simulink model "Cooperative_Localization_05_New2"  (R2016b)
settings: Solver=ode45  StartTime=0.0  StopTime=200  RelTol=1e-3  EnableMultiTasking=on
InitFcn:
  | Const_Coop_Local_05
undefined symbols (not defined in the file): alpha, AN, B, B_pseudo_inverse, BBT_inv, BN, D, Delta_form, Gama0, gamma0, gamma_0, gamma_1, H, K, k0_est, k1, k1_est, k2, KI, Ki_1, Ki_2, Ki_3, Ki_4, lambda, m_cont, Mb, Mu, n, N, n_cont, Observer_Gain, P_struct, Q, Q1, R, Rho1, Rho_0, rho_0, rho_1, t_cont, U_dot0_M
(part 1 of 3)
settings Model: SimulationMode=rapid-accelerator  Creator=hp  LastModifiedBy=hp
settings DataIOCC: LimitDataPoints=on  SaveFormat=Array
settings OptimizationCC: LifeSpan=inf
settings DebuggingCC: UnderspecifiedInitializationDetection=Classic  MergeDetectMultiDrivingBlocksExec=none  SolverPrmCheckMsg=warning  SFUnexpectedBacktrackingDiag=warning  SFNoUnconditionalDefaultTransitionDiag=warning  SFExecutionAtInitializationDiag=none
settings HardwareCC: ProdBitPerPointer=32  ProdBitPerSizeT=32  ProdBitPerPtrDiffT=32  ProdLargestAtomicFloat=None  ProdIntDivRoundTo=Undefined  ProdEndianess=Unspecified  ProdWordSize=32  ProdHWDeviceType=32-bit Generic
settings ModelReferenceCC: PropagateSignalLabelsOutOfModel=off
settings GRTTargetCC: TargetLangStandard=C89/C90 (ANSI)  GeneratePreprocessorConditionals=Disable all
settings ConfigComp: CovMetricSettings=dw  CovHtmlReporting=on  CovSaveCumulativeToWorkspaceVar=on  CovSaveSingleToWorkspaceVar=on  CovExternalEMLEnable=off

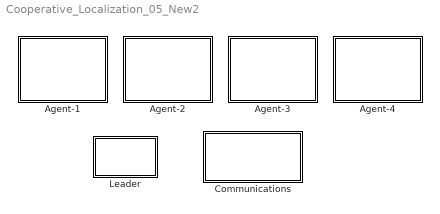
== system Cooperative_Localization_05_New2 ==
  Agent-1 : Subsystem
  Agent-2 : Subsystem
  Agent-3 : Subsystem
  Agent-4 : Subsystem
  Communications : Subsystem
  Leader : Subsystem

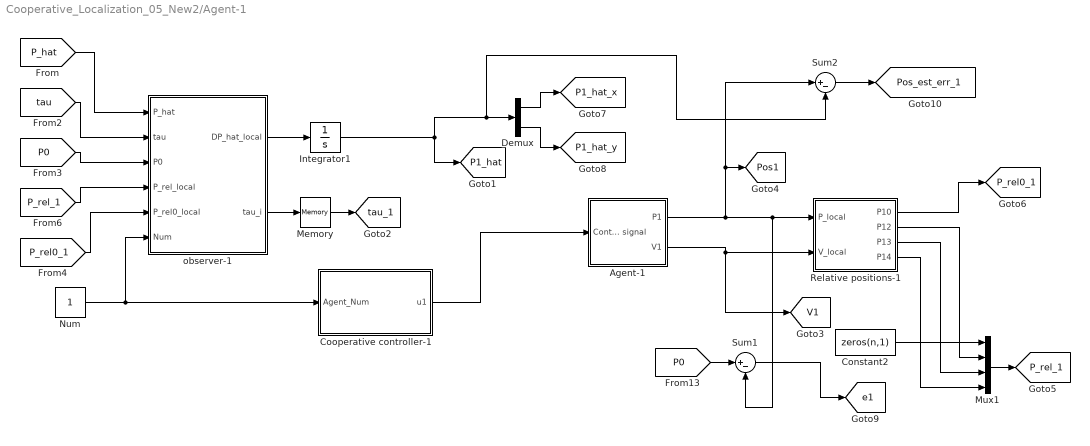
== system Cooperative_Localization_05_New2/Agent-1 ==
  Agent-1 : Subsystem
  Constant2 : Constant  Value=zeros(n,1)
  Cooperative controller-1 : Subsystem
  Demux : Demux  Outputs=2
  Integrator1 : Integrator  InitialCondition=zeros(n,1)
  Memory : Memory  X0=zeros(n,1)
  Mux1 : Mux
  Num : Constant
  Relative positions-1 : Subsystem
  Sum1 : Sum  Inputs=|+-
  Sum2 : Sum  Inputs=|+-
  observer-1 : MATLAB Function  TreatAsAtomicUnit=on
  tag scope: P1_hat=global, P1_hat_x=global, P1_hat_y=global, P_rel0_1=global, P_rel_1=global, Pos1=global, Pos_est_err_1=global, V1=global, e1=global, tau_1=global
  wires:
  observer-1/1(DP_hat_local) -> Integrator1/1
  Integrator1/1 -> [P1_hat], Sum2/2, Demux/1
  [P_hat] -> observer-1/1(P_hat)
  [tau] -> observer-1/2(tau)
  [P0] -> observer-1/3(P0)
  [P_rel0_1] -> observer-1/5(P_rel0_local)
  observer-1/2(tau_i) -> Memory/1
  [P_rel_1] -> observer-1/4(P_rel_local)
  Memory/1 -> [tau_1]
  Agent-1/2(V1) -> Relative positions-1/2(V_local), [V1]
  Agent-1/1(P1) -> Relative positions-1/1(P_local), Sum1/2, [Pos1], Sum2/1
  Mux1/1 -> [P_rel_1]
  Relative positions-1/1(P10) -> [P_rel0_1]
  Demux/1 -> [P1_hat_x]
  Demux/2 -> [P1_hat_y]
  Constant2/1 -> Mux1/1
  Relative positions-1/2(P12) -> Mux1/2
  Relative positions-1/3(P13) -> Mux1/3
  Relative positions-1/4(P14) -> Mux1/4
  Sum1/1 -> [e1]
  Sum2/1 -> [Pos_est_err_1]
  [P0] -> Sum1/1
  Num/1 -> Cooperative controller-1/1(Agent_Num), observer-1/6(Num)
  Cooperative controller-1/1(u1) -> Agent-1/1(Control signal)

== system Cooperative_Localization_05_New2/Agent-2 ==
  Agent-2 : Subsystem
  Constant2 : Constant  Value=zeros(n,1)
  Cooperative controller-2 : Subsystem
  Demux : Demux  Outputs=2
  Integrator1 : Integrator  InitialCondition=zeros(n,1)
  Memory : Memory  X0=zeros(n,1)
  Mux1 : Mux
  Num : Constant  Value=2
  Relative positions-2 : Subsystem
  Sum1 : Sum  Inputs=|+-
  Sum2 : Sum  Inputs=|+-
  observer-1 : MATLAB Function  TreatAsAtomicUnit=on
  tag scope: P2_hat=global, P2_hat_x=global, P2_hat_y=global, P_rel0_2=global, P_rel_2=global, Pos2=global, Pos_est_err_2=global, V2=global, e2=global, tau_2=global
  wires:
  Relative positions-2/4(P24) -> Mux1/4
  Relative positions-2/3(P23) -> Mux1/3
  Demux/2 -> [P2_hat_y]
  Demux/1 -> [P2_hat_x]
  Relative positions-2/1(P20) -> [P_rel0_2]
  Mux1/1 -> [P_rel_2]
  Agent-2/2(V2) -> Relative positions-2/2(V_local), [V2]
  Cooperative controller-2/1(u2) -> Agent-2/1(Control signal)
  Memory/1 -> [tau_2]
  [P_rel_2] -> observer-1/4(P_rel_local)
  observer-1/2(tau_i) -> Memory/1
  [P_rel0_2] -> observer-1/5(P_rel0_local)
  [P0] -> observer-1/3(P0)
  [tau] -> observer-1/2(tau)
  [P_hat] -> observer-1/1(P_hat)
  observer-1/1(DP_hat_local) -> Integrator1/1
  Constant2/1 -> Mux1/2
  Relative positions-2/2(P21) -> Mux1/1
  Sum1/1 -> [e2]
  Integrator1/1 -> Sum2/2, Demux/1, [P2_hat]
  Agent-2/1(P2) -> Sum2/1, [Pos2], Relative positions-2/1(P_local), Sum1/2
  Sum2/1 -> [Pos_est_err_2]
  Num/1 -> Cooperative controller-2/1(Agent_Num), observer-1/6(Num)
  [P0] -> Sum1/1

== system Cooperative_Localization_05_New2/Agent-3 ==
  Agent-3 : Subsystem
  Constant2 : Constant  Value=zeros(n,1)
  Cooperative controller-3 : Subsystem
  Demux : Demux  Outputs=2
  Integrator1 : Integrator  InitialCondition=zeros(n,1)
  Memory : Memory  X0=zeros(n,1)
  Mux1 : Mux
  Num : Constant  Value=3
  Relative positions-3 : Subsystem
  Sum1 : Sum  Inputs=|+-
  Sum2 : Sum  Inputs=|+-
  observer-1 : MATLAB Function  TreatAsAtomicUnit=on
  tag scope: P3_hat=global, P3_hat_x=global, P3_hat_y=global, P_rel0_3=global, P_rel_3=global, Pos3=global, Pos_est_err_3=global, V3=global, e3=global, tau_3=global
  wires:
  observer-1/1(DP_hat_local) -> Integrator1/1
  [P_hat] -> observer-1/1(P_hat)
  [tau] -> observer-1/2(tau)
  [P0] -> observer-1/3(P0)
  [P_rel0_3] -> observer-1/5(P_rel0_local)
  observer-1/2(tau_i) -> Memory/1
  [P_rel_3] -> observer-1/4(P_rel_local)
  Memory/1 -> [tau_3]
  Agent-3/2(V3) -> Relative positions-3/2(V_local), [V3]
  Mux1/1 -> [P_rel_3]
  Relative positions-3/1(P30) -> [P_rel0_3]
  Demux/1 -> [P3_hat_x]
  Demux/2 -> [P3_hat_y]
  Constant2/1 -> Mux1/3
  Relative positions-3/2(P31) -> Mux1/1
  Relative positions-3/3(P32) -> Mux1/2
  Relative positions-3/4(P34) -> Mux1/4
  Sum1/1 -> [e3]
  Integrator1/1 -> [P3_hat], Sum2/2, Demux/1
  Agent-3/1(P3) -> Relative positions-3/1(P_local), Sum1/2, Sum2/1, [Pos3]
  Sum2/1 -> [Pos_est_err_3]
  Num/1 -> Cooperative controller-3/1(Agent_Num), observer-1/6(Num)
  [P0] -> Sum1/1
  Cooperative controller-3/1(u3) -> Agent-3/1(Control signal)

== system Cooperative_Localization_05_New2/Agent-4 ==
  Agent-4 : Subsystem
  Constant2 : Constant  Value=zeros(n,1)
  Cooperative controller-4 : Subsystem
  Demux : Demux  Outputs=2
  Integrator1 : Integrator  InitialCondition=zeros(n,1)
  Memory : Memory  X0=zeros(n,1)
  Mux1 : Mux
  Num : Constant  Value=4
  Relative positions-4 : Subsystem
  Sum1 : Sum  Inputs=|+-
  Sum2 : Sum  Inputs=|+-
  observer-1 : MATLAB Function  TreatAsAtomicUnit=on
  tag scope: P4_hat=global, P4_hat_x=global, P4_hat_y=global, P_rel0_4=global, P_rel_4=global, Pos4=global, Pos_est_err_4=global, V4=global, e4=global, tau_4=global
  wires:
  Demux/2 -> [P4_hat_y]
  Demux/1 -> [P4_hat_x]
  Relative positions-4/1(P40) -> [P_rel0_4]
  Mux1/1 -> [P_rel_4]
  Agent-4/2(V4) -> Relative positions-4/2(V_local), [V4]
  Memory/1 -> [tau_4]
  [P_rel_4] -> observer-1/4(P_rel_local)
  observer-1/2(tau_i) -> Memory/1
  [P_rel0_4] -> observer-1/5(P_rel0_local)
  [P0] -> observer-1/3(P0)
  [tau] -> observer-1/2(tau)
  [P_hat] -> observer-1/1(P_hat)
  observer-1/1(DP_hat_local) -> Integrator1/1
  Constant2/1 -> Mux1/4
  Relative positions-4/2(P41) -> Mux1/1
  Relative positions-4/3(P42) -> Mux1/2
  Relative positions-4/4(P43) -> Mux1/3
  Sum1/1 -> [e4]
  Integrator1/1 -> Sum2/2, Demux/1, [P4_hat]
  Agent-4/1(P4) -> Sum2/1, [Pos4], Relative positions-4/1(P_local), Sum1/2
  Sum2/1 -> [Pos_est_err_4]
  Num/1 -> Cooperative controller-4/1(Agent_Num), observer-1/6(Num)
  [P0] -> Sum1/1
  Cooperative controller-4/1(u4) -> Agent-4/1(Control signal)

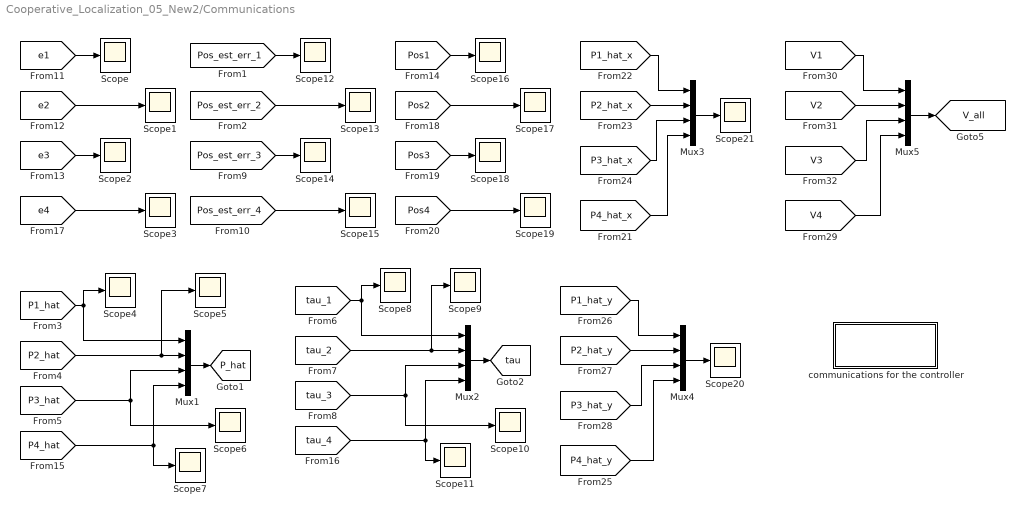
== system Cooperative_Localization_05_New2/Communications ==
  Mux{1..5} (5 alike) : Mux
  Scope{,1..21} (22 alike) : Scope
  communications for the controller : Subsystem
  tag scope: P_hat=global, V_all=global, tau=global
  wires:
  [P1_hat] -> Scope4/1, Mux1/1
  [P2_hat] -> Scope5/1, Mux1/2
  [P3_hat] -> Mux1/3, Scope6/1
  Mux1/1 -> [P_hat]
  [tau_1] -> Scope8/1, Mux2/1
  [tau_2] -> Scope9/1, Mux2/2
  [tau_3] -> Mux2/3, Scope10/1
  Mux2/1 -> [tau]
  [P4_hat] -> Scope7/1, Mux1/4
  [tau_4] -> Scope11/1, Mux2/4
  [e1] -> Scope/1
  [e2] -> Scope1/1
  [e3] -> Scope2/1
  [e4] -> Scope3/1
  [Pos_est_err_1] -> Scope12/1
  [Pos_est_err_2] -> Scope13/1
  [Pos_est_err_3] -> Scope14/1
  [Pos_est_err_4] -> Scope15/1
  [Pos1] -> Scope16/1
  [Pos2] -> Scope17/1
  [Pos3] -> Scope18/1
  [Pos4] -> Scope19/1
  [P1_hat_x] -> Mux3/1
  [P2_hat_x] -> Mux3/2
  [P3_hat_x] -> Mux3/3
  Mux3/1 -> Scope21/1
  [P4_hat_x] -> Mux3/4
  [P1_hat_y] -> Mux4/1
  [P2_hat_y] -> Mux4/2
  [P3_hat_y] -> Mux4/3
  Mux4/1 -> Scope20/1
  [P4_hat_y] -> Mux4/4
  [V1] -> Mux5/1
  [V2] -> Mux5/2
  [V3] -> Mux5/3
  Mux5/1 -> [V_all]
  [V4] -> Mux5/4

== system Cooperative_Localization_05_New2/Leader ==
  Agent-0 : Subsystem
  Ali : Subsystem
  Constant4 : Constant  Value=2
  Constant5 : Constant
  Controller interpreter : MATLAB Function  TreatAsAtomicUnit=on
  Mux1 : Mux  Inputs=2
  Mux2 : Mux  Inputs=2
  Scope{,1..4} (5 alike) : Scope
  Sine Wave : Sin  Amplitude=4  Frequency=0.1  SampleTime=0
  Sine Wave1 : Sin  Amplitude=6  Frequency=0.05  SampleTime=0
  Sum : Sum  Inputs=|+-
  Transfer Fcn : TransferFcn  Denominator=[10 1]
  Transfer Fcn1 : TransferFcn  Denominator=[10 1]
  formation of the leader : Constant  Value=zeros(n_cont,1)
  tag scope: P0=global, U0=global, V0=global, Z0=global
  wires:
  Sum/1 -> [Z0]
  formation of the leader/1 -> Sum/2
  Controller interpreter/1(u) -> Agent-0/1(Control signal), Mux2/2
  Ali/1(u) -> Scope/1, Controller interpreter/1(U)
  Mux1/1 -> Ali/2(xd), Scope4/1
  Constant4/1 -> Transfer Fcn/1
  Constant5/1 -> Transfer Fcn1/1
  Agent-0/2(P0) -> [P0], Scope1/1
  Mux2/1 -> [U0]
  Agent-0/1(X0) -> Ali/1(x), Scope2/1, Sum/1
  Agent-0/3(V0) -> Scope3/1, Mux2/1, [V0]
  Sine Wave/1 -> Mux1/1
  Sine Wave1/1 -> Mux1/2

== system Cooperative_Localization_05_New2/Agent-1/Agent-1 ==
  Control signal : Inport
  Clock : Clock
  Demux : Demux
  Demux1 : Demux  Outputs=2
  Integrator : Integrator  InitialCondition=[0;0;0;0]
  MATLAB Function : MATLAB Function  TreatAsAtomicUnit=on
  Memory1 : Memory  X0=zeros(2,1)
  Memory4 : Memory  X0=zeros(2,1)
  Mux : Mux  Inputs=2
  Mux1 : Mux  Inputs=2
  P1 : Outport
  V1 : Outport  Port=2
  wires:
  MATLAB Function/1(out) -> Integrator/1
  Integrator/1 -> Demux/1
  Mux/1 -> Memory4/1
  Mux1/1 -> Memory1/1
  Control signal/1 -> Demux1/1
  Demux1/1 -> MATLAB Function/5(Ax)
  Demux1/2 -> MATLAB Function/6(Ay)
  Memory4/1 -> P1/1
  Memory1/1 -> V1/1
  Demux/3 -> MATLAB Function/3(Vx), Mux1/1
  Demux/4 -> MATLAB Function/4(Vy), Mux1/2
  Demux/1 -> MATLAB Function/1(Px), Mux/1
  Demux/2 -> MATLAB Function/2(Py), Mux/2
  Clock/1 -> MATLAB Function/7(t)

== system Cooperative_Localization_05_New2/Agent-1/Cooperative controller-1 ==
  Agent_Num : Inport
  Choosing real control variables : MATLAB Function  TreatAsAtomicUnit=on
  Decenteralized Cooperaive Controller #1 : Subsystem
  Module to compute Consensus Error #1 : MATLAB Function  TreatAsAtomicUnit=on
  Mux : Mux  Inputs=2
  Variable change : MATLAB Function  TreatAsAtomicUnit=on
  u1 : Outport
  tag scope: E1_Cont=global, X1_Cont=global
  wires:
  Agent_Num/1 -> Module to compute Consensus Error #1/6(Agent_Num), Decenteralized Cooperaive Controller #1/1(Agent #)
  Decenteralized Cooperaive Controller #1/1(U1) -> Variable change/1(U), Choosing real control variables/1(U)
  [P_rel0_1] -> Module to compute Consensus Error #1/2(P_rel0)
  Module to compute Consensus Error #1/1(Ep) -> [E1_Cont]
  [P_rel_1] -> Module to compute Consensus Error #1/1(P_rel_all)
  Choosing real control variables/1(u) -> u1/1
  Variable change/1(X_mod) -> [X1_Cont]
  Mux/1 -> Variable change/2(X)
  [P1_hat] -> Mux/1
  [V1] -> Mux/2
  [V1] -> Module to compute Consensus Error #1/3(V_loc)
  [V0] -> Module to compute Consensus Error #1/4(V0)
  [V_all] -> Module to compute Consensus Error #1/5(V_all)

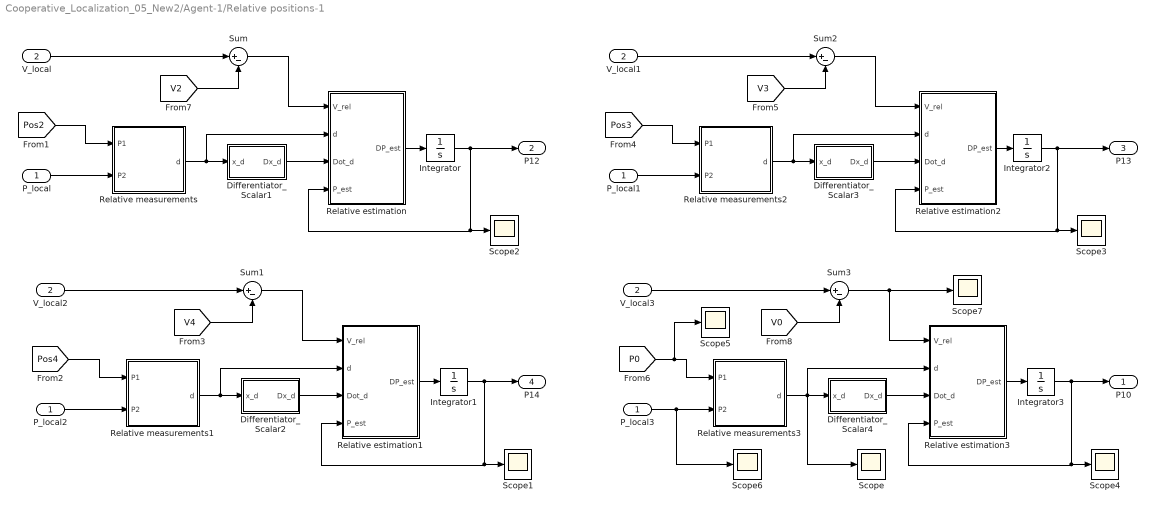
== system Cooperative_Localization_05_New2/Agent-1/Relative positions-1 ==
  P_local : Inport
  V_local : Inport  Port=2
  Differentiator_Scalar1 : Subsystem
  Differentiator_Scalar2 : Subsystem
  Differentiator_Scalar3 : Subsystem
  Differentiator_Scalar4 : Subsystem
  Integrator{,1..3} (4 alike) : Integrator  InitialCondition=zeros(2,1)
  P_local1 : InportShadow
  P_local2 : InportShadow
  P_local3 : InportShadow
  Relative estimation : MATLAB Function  TreatAsAtomicUnit=on
  Relative estimation1 : MATLAB Function  TreatAsAtomicUnit=on
  Relative estimation2 : MATLAB Function  TreatAsAtomicUnit=on
  Relative estimation3 : MATLAB Function  TreatAsAtomicUnit=on
  Relative measurements : MATLAB Function  TreatAsAtomicUnit=on
  Relative measurements1 : MATLAB Function  TreatAsAtomicUnit=on
  Relative measurements2 : MATLAB Function  TreatAsAtomicUnit=on
  Relative measurements3 : MATLAB Function  TreatAsAtomicUnit=on
  Scope{,1..7} (8 alike) : Scope
  Sum{,1..3} (4 alike) : Sum  Inputs=|+-
  V_local1 : InportShadow  Port=2
  V_local2 : InportShadow  Port=2
  V_local3 : InportShadow  Port=2
  P10 : Outport
  P12 : Outport  Port=2
  P13 : Outport  Port=3
  P14 : Outport  Port=4
  wires:
  Relative measurements/1(d) -> Relative estimation/2(d), Differentiator_Scalar1/1(x_d)
  Differentiator_Scalar1/1(Dx_d) -> Relative estimation/3(Dot_d)
  Relative estimation/1(DP_est) -> Integrator/1
  Integrator/1 -> P12/1, Scope2/1, Relative estimation/4(P_est)
  P_local/1 -> Relative measurements/2(P2)
  V_local/1 -> Sum/1
  Sum/1 -> Relative estimation/1(V_rel)
  [V2] -> Sum/2
  [Pos2] -> Relative measurements/1(P1)
  Relative measurements1/1(d) -> Relative estimation1/2(d), Differentiator_Scalar2/1(x_d)
  Differentiator_Scalar2/1(Dx_d) -> Relative estimation1/3(Dot_d)
  Relative estimation1/1(DP_est) -> Integrator1/1
  Integrator1/1 -> P14/1, Relative estimation1/4(P_est), Scope1/1
  P_local2/1 -> Relative measurements1/2(P2)
  V_local2/1 -> Sum1/1
  Sum1/1 -> Relative estimation1/1(V_rel)
  [V4] -> Sum1/2
  [Pos4] -> Relative measurements1/1(P1)
  Relative measurements2/1(d) -> Relative estimation2/2(d), Differentiator_Scalar3/1(x_d)
  Differentiator_Scalar3/1(Dx_d) -> Relative estimation2/3(Dot_d)
  Relative estimation2/1(DP_est) -> Integrator2/1
  Integrator2/1 -> P13/1, Relative estimation2/4(P_est), Scope3/1
  P_local1/1 -> Relative measurements2/2(P2)
  V_local1/1 -> Sum2/1
  Sum2/1 -> Relative estimation2/1(V_rel)
  [V3] -> Sum2/2
  [Pos3] -> Relative measurements2/1(P1)
  Relative measurements3/1(d) -> Scope/1, Relative estimation3/2(d), Differentiator_Scalar4/1(x_d)
  Differentiator_Scalar4/1(Dx_d) -> Relative estimation3/3(Dot_d)
  Relative estimation3/1(DP_est) -> Integrator3/1
  Integrator3/1 -> P10/1, Relative estimation3/4(P_est), Scope4/1
  P_local3/1 -> Scope6/1, Relative measurements3/2(P2)
  V_local3/1 -> Sum3/1
  Sum3/1 -> Scope7/1, Relative estimation3/1(V_rel)
  [V0] -> Sum3/2
  [P0] -> Scope5/1, Relative measurements3/1(P1)

== system Cooperative_Localization_05_New2/Agent-2/Agent-2 ==
  Control signal : Inport
  Clock : Clock
  Demux : Demux
  Demux1 : Demux  Outputs=2
  Integrator : Integrator  InitialCondition=[0;0;0;0]
  MATLAB Function : MATLAB Function  TreatAsAtomicUnit=on
  Memory1 : Memory  X0=zeros(2,1)
  Memory4 : Memory  X0=zeros(2,1)
  Mux : Mux  Inputs=2
  Mux1 : Mux  Inputs=2
  P2 : Outport
  V2 : Outport  Port=2
  wires:
  Demux/2 -> MATLAB Function/2(Py), Mux/2
  Demux/1 -> MATLAB Function/1(Px), Mux/1
  Demux/4 -> MATLAB Function/4(Vy), Mux1/2
  Demux/3 -> MATLAB Function/3(Vx), Mux1/1
  Memory1/1 -> V2/1
  Memory4/1 -> P2/1
  Demux1/2 -> MATLAB Function/6(Ay)
  Demux1/1 -> MATLAB Function/5(Ax)
  Control signal/1 -> Demux1/1
  Mux1/1 -> Memory1/1
  Mux/1 -> Memory4/1
  Integrator/1 -> Demux/1
  MATLAB Function/1(out) -> Integrator/1
  Clock/1 -> MATLAB Function/7(t)

== system Cooperative_Localization_05_New2/Agent-2/Cooperative controller-2 ==
  Agent_Num : Inport
  Choosing real control variables : MATLAB Function  TreatAsAtomicUnit=on
  Decenteralized Cooperaive Controller #2 : Subsystem
  Module to compute Consensus Error #2 : MATLAB Function  TreatAsAtomicUnit=on
  Mux : Mux  Inputs=2
  Variable change : MATLAB Function  TreatAsAtomicUnit=on
  u2 : Outport
  tag scope: E2_Cont=global, X2_Cont=global
  wires:
  Agent_Num/1 -> Module to compute Consensus Error #2/6(Agent_Num), Decenteralized Cooperaive Controller #2/1(Agent #)
  Decenteralized Cooperaive Controller #2/1(U2) -> Variable change/1(U), Choosing real control variables/1(U)
  [P_rel0_2] -> Module to compute Consensus Error #2/2(P_rel0)
  Module to compute Consensus Error #2/1(Ep) -> [E2_Cont]
  [P_rel_2] -> Module to compute Consensus Error #2/1(P_rel_all)
  Choosing real control variables/1(u) -> u2/1
  Variable change/1(X_mod) -> [X2_Cont]
  Mux/1 -> Variable change/2(X)
  [P2_hat] -> Mux/1
  [V2] -> Mux/2
  [V2] -> Module to compute Consensus Error #2/3(V_loc)
  [V0] -> Module to compute Consensus Error #2/4(V0)
  [V_all] -> Module to compute Consensus Error #2/5(V_all)

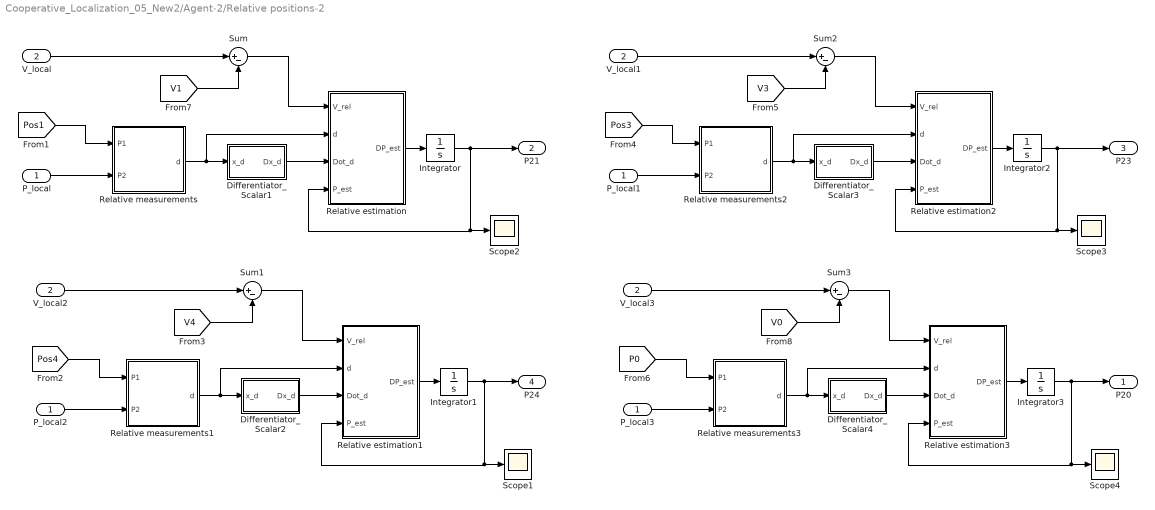
== system Cooperative_Localization_05_New2/Agent-2/Relative positions-2 ==
  P_local : Inport
  V_local : Inport  Port=2
  Differentiator_Scalar1 : Subsystem
  Differentiator_Scalar2 : Subsystem
  Differentiator_Scalar3 : Subsystem
  Differentiator_Scalar4 : Subsystem
  Integrator{,1..3} (4 alike) : Integrator  InitialCondition=zeros(2,1)
  P_local1 : InportShadow
  P_local2 : InportShadow
  P_local3 : InportShadow
  Relative estimation : MATLAB Function  TreatAsAtomicUnit=on
  Relative estimation1 : MATLAB Function  TreatAsAtomicUnit=on
  Relative estimation2 : MATLAB Function  TreatAsAtomicUnit=on
  Relative estimation3 : MATLAB Function  TreatAsAtomicUnit=on
  Relative measurements : MATLAB Function  TreatAsAtomicUnit=on
  Relative measurements1 : MATLAB Function  TreatAsAtomicUnit=on
  Relative measurements2 : MATLAB Function  TreatAsAtomicUnit=on
  Relative measurements3 : MATLAB Function  TreatAsAtomicUnit=on
  Scope{1..4} (4 alike) : Scope
  Sum{,1..3} (4 alike) : Sum  Inputs=|+-
  V_local1 : InportShadow  Port=2
  V_local2 : InportShadow  Port=2
  V_local3 : InportShadow  Port=2
  P20 : Outport
  P21 : Outport  Port=2
  P23 : Outport  Port=3
  P24 : Outport  Port=4
  wires:
  [P0] -> Relative measurements3/1(P1)
  [V0] -> Sum3/2
  Sum3/1 -> Relative estimation3/1(V_rel)
  V_local3/1 -> Sum3/1
  P_local3/1 -> Relative measurements3/2(P2)
  Integrator3/1 -> Relative estimation3/4(P_est), Scope4/1, P20/1
  Relative estimation3/1(DP_est) -> Integrator3/1
  Differentiator_Scalar4/1(Dx_d) -> Relative estimation3/3(Dot_d)
  Relative measurements3/1(d) -> Relative estimation3/2(d), Differentiator_Scalar4/1(x_d)
  [Pos3] -> Relative measurements2/1(P1)
  [V3] -> Sum2/2
  Sum2/1 -> Relative estimation2/1(V_rel)
  V_local1/1 -> Sum2/1
  P_local1/1 -> Relative measurements2/2(P2)
  Integrator2/1 -> Relative estimation2/4(P_est), Scope3/1, P23/1
  Relative estimation2/1(DP_est) -> Integrator2/1
  Differentiator_Scalar3/1(Dx_d) -> Relative estimation2/3(Dot_d)
  Relative measurements2/1(d) -> Relative estimation2/2(d), Differentiator_Scalar3/1(x_d)
  [Pos4] -> Relative measurements1/1(P1)
  [V4] -> Sum1/2
  Sum1/1 -> Relative estimation1/1(V_rel)
  V_local2/1 -> Sum1/1
  P_local2/1 -> Relative measurements1/2(P2)
  Integrator1/1 -> Relative estimation1/4(P_est), Scope1/1, P24/1
  Relative estimation1/1(DP_est) -> Integrator1/1
  Differentiator_Scalar2/1(Dx_d) -> Relative estimation1/3(Dot_d)
  Relative measurements1/1(d) -> Relative estimation1/2(d), Differentiator_Scalar2/1(x_d)
  [Pos1] -> Relative measurements/1(P1)
  [V1] -> Sum/2
  Sum/1 -> Relative estimation/1(V_rel)
  V_local/1 -> Sum/1
  P_local/1 -> Relative measurements/2(P2)
  Integrator/1 -> Relative estimation/4(P_est), Scope2/1, P21/1
  Relative estimation/1(DP_est) -> Integrator/1
  Differentiator_Scalar1/1(Dx_d) -> Relative estimation/3(Dot_d)
  Relative measurements/1(d) -> Relative estimation/2(d), Differentiator_Scalar1/1(x_d)

== system Cooperative_Localization_05_New2/Agent-3/Agent-3 ==
  Control signal : Inport
  Clock : Clock
  Demux : Demux
  Demux1 : Demux  Outputs=2
  Integrator : Integrator  InitialCondition=[0;0;0;0]
  MATLAB Function : MATLAB Function  TreatAsAtomicUnit=on
  Memory1 : Memory  X0=zeros(2,1)
  Memory4 : Memory  X0=[0;0]
  Mux : Mux  Inputs=2
  Mux1 : Mux  Inputs=2
  P3 : Outport
  V3 : Outport  Port=2
  tag scope: Vx3=global, Vy3=global
  wires:
  MATLAB Function/1(out) -> Integrator/1
  Integrator/1 -> Demux/1
  Mux/1 -> Memory4/1
  Mux1/1 -> Memory1/1
  Control signal/1 -> Demux1/1
  Demux1/1 -> MATLAB Function/5(Ax)
  Demux1/2 -> MATLAB Function/6(Ay)
  Memory4/1 -> P3/1
  Memory1/1 -> V3/1
  Demux/3 -> MATLAB Function/3(Vx), [Vx3], Mux1/1
  Demux/4 -> MATLAB Function/4(Vy), [Vy3], Mux1/2
  Demux/1 -> MATLAB Function/1(Px), Mux/1
  Demux/2 -> MATLAB Function/2(Py), Mux/2
  Clock/1 -> MATLAB Function/7(t)

== system Cooperative_Localization_05_New2/Agent-3/Cooperative controller-3 ==
  Agent_Num : Inport
  Choosing real control variables : MATLAB Function  TreatAsAtomicUnit=on
  Decenteralized Cooperaive Controller #3 : Subsystem
  Module to compute Consensus Error #3 : MATLAB Function  TreatAsAtomicUnit=on
  Mux : Mux  Inputs=2
  Variable change : MATLAB Function  TreatAsAtomicUnit=on
  u3 : Outport
  tag scope: E3_Cont=global, X3_Cont=global
  wires:
  Agent_Num/1 -> Module to compute Consensus Error #3/6(Agent_Num), Decenteralized Cooperaive Controller #3/1(Agent #)
  Decenteralized Cooperaive Controller #3/1(U3) -> Variable change/1(U), Choosing real control variables/1(U)
  [P_rel0_3] -> Module to compute Consensus Error #3/2(P_rel0)
  Module to compute Consensus Error #3/1(Ep) -> [E3_Cont]
  [P_rel_3] -> Module to compute Consensus Error #3/1(P_rel_all)
  Choosing real control variables/1(u) -> u3/1
  Variable change/1(X_mod) -> [X3_Cont]
  Mux/1 -> Variable change/2(X)
  [P3_hat] -> Mux/1
  [V3] -> Mux/2
  [V3] -> Module to compute Consensus Error #3/3(V_loc)
  [V0] -> Module to compute Consensus Error #3/4(V0)
  [V_all] -> Module to compute Consensus Error #3/5(V_all)

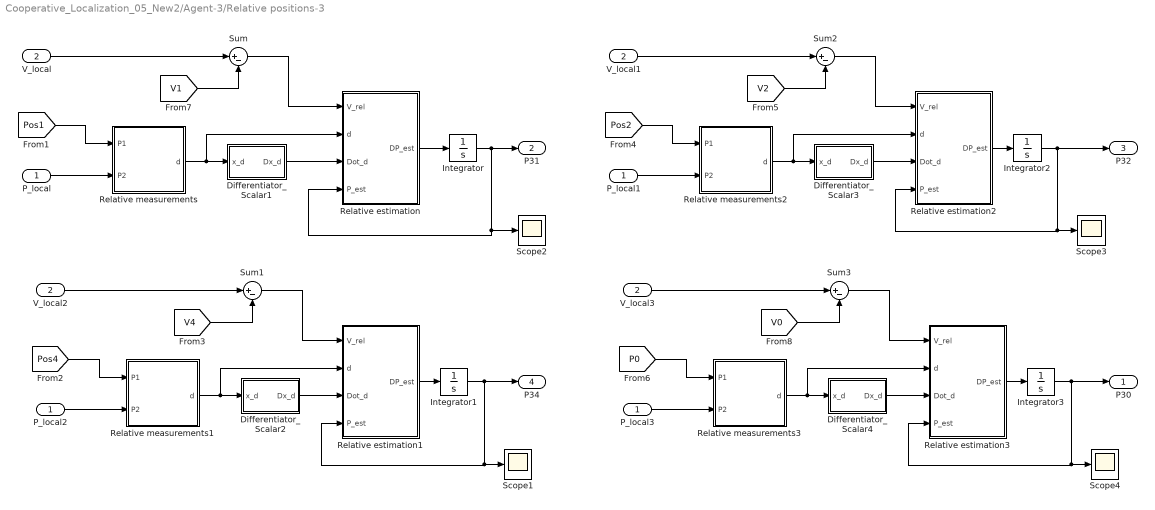
== system Cooperative_Localization_05_New2/Agent-3/Relative positions-3 ==
  P_local : Inport
  V_local : Inport  Port=2
  Differentiator_Scalar1 : Subsystem
  Differentiator_Scalar2 : Subsystem
  Differentiator_Scalar3 : Subsystem
  Differentiator_Scalar4 : Subsystem
  Integrator{,1..3} (4 alike) : Integrator  InitialCondition=zeros(2,1)
  P_local1 : InportShadow
  P_local2 : InportShadow
  P_local3 : InportShadow
  Relative estimation : MATLAB Function  TreatAsAtomicUnit=on
  Relative estimation1 : MATLAB Function  TreatAsAtomicUnit=on
  Relative estimation2 : MATLAB Function  TreatAsAtomicUnit=on
  Relative estimation3 : MATLAB Function  TreatAsAtomicUnit=on
  Relative measurements : MATLAB Function  TreatAsAtomicUnit=on
  Relative measurements1 : MATLAB Function  TreatAsAtomicUnit=on
  Relative measurements2 : MATLAB Function  TreatAsAtomicUnit=on
  Relative measurements3 : MATLAB Function  TreatAsAtomicUnit=on
  Scope{1..4} (4 alike) : Scope
  Sum{,1..3} (4 alike) : Sum  Inputs=|+-
  V_local1 : InportShadow  Port=2
  V_local2 : InportShadow  Port=2
  V_local3 : InportShadow  Port=2
  P30 : Outport
  P31 : Outport  Port=2
  P32 : Outport  Port=3
  P34 : Outport  Port=4
  wires:
  Relative measurements/1(d) -> Relative estimation/2(d), Differentiator_Scalar1/1(x_d)
  Differentiator_Scalar1/1(Dx_d) -> Relative estimation/3(Dot_d)
  Relative estimation/1(DP_est) -> Integrator/1
  Integrator/1 -> P31/1, Relative estimation/4(P_est), Scope2/1
  P_local/1 -> Relative measurements/2(P2)
  V_local/1 -> Sum/1
  Sum/1 -> Relative estimation/1(V_rel)
  [V1] -> Sum/2
  [Pos1] -> Relative measurements/1(P1)
  Relative measurements1/1(d) -> Relative estimation1/2(d), Differentiator_Scalar2/1(x_d)
  Differentiator_Scalar2/1(Dx_d) -> Relative estimation1/3(Dot_d)
  Relative estimation1/1(DP_est) -> Integrator1/1
  Integrator1/1 -> P34/1, Relative estimation1/4(P_est), Scope1/1
  P_local2/1 -> Relative measurements1/2(P2)
  V_local2/1 -> Sum1/1
  Sum1/1 -> Relative estimation1/1(V_rel)
  [V4] -> Sum1/2
  [Pos4] -> Relative measurements1/1(P1)
  Relative measurements2/1(d) -> Relative estimation2/2(d), Differentiator_Scalar3/1(x_d)
  Differentiator_Scalar3/1(Dx_d) -> Relative estimation2/3(Dot_d)
  Relative estimation2/1(DP_est) -> Integrator2/1
  Integrator2/1 -> P32/1, Relative estimation2/4(P_est), Scope3/1
  P_local1/1 -> Relative measurements2/2(P2)
  V_local1/1 -> Sum2/1
  Sum2/1 -> Relative estimation2/1(V_rel)
  [V2] -> Sum2/2
  [Pos2] -> Relative measurements2/1(P1)
  Relative measurements3/1(d) -> Relative estimation3/2(d), Differentiator_Scalar4/1(x_d)
  Differentiator_Scalar4/1(Dx_d) -> Relative estimation3/3(Dot_d)
  Relative estimation3/1(DP_est) -> Integrator3/1
  Integrator3/1 -> P30/1, Relative estimation3/4(P_est), Scope4/1
  P_local3/1 -> Relative measurements3/2(P2)
  V_local3/1 -> Sum3/1
  Sum3/1 -> Relative estimation3/1(V_rel)
  [V0] -> Sum3/2
  [P0] -> Relative measurements3/1(P1)

== system Cooperative_Localization_05_New2/Agent-4/Agent-4 ==
  Control signal : Inport
  Clock : Clock
  Demux : Demux
  Demux1 : Demux  Outputs=2
  Integrator : Integrator  InitialCondition=[0;0;0;0]
  MATLAB Function : MATLAB Function  TreatAsAtomicUnit=on
  Memory1 : Memory  X0=zeros(2,1)
  Memory4 : Memory  X0=zeros(2,1)
  Mux : Mux  Inputs=2
  Mux1 : Mux  Inputs=2
  P4 : Outport
  V4 : Outport  Port=2
  tag scope: Vx4=global, Vy4=global
  wires:
  Demux/2 -> MATLAB Function/2(Py), Mux/2
  Demux/1 -> MATLAB Function/1(Px), Mux/1
  Demux/4 -> MATLAB Function/4(Vy), Mux1/2, [Vy4]
  Demux/3 -> MATLAB Function/3(Vx), Mux1/1, [Vx4]
  Memory1/1 -> V4/1
  Memory4/1 -> P4/1
  Demux1/2 -> MATLAB Function/6(Ay)
  Demux1/1 -> MATLAB Function/5(Ax)
  Control signal/1 -> Demux1/1
  Mux1/1 -> Memory1/1
  Mux/1 -> Memory4/1
  Integrator/1 -> Demux/1
  MATLAB Function/1(out) -> Integrator/1
  Clock/1 -> MATLAB Function/7(t)

== system Cooperative_Localization_05_New2/Agent-4/Cooperative controller-4 ==
  Agent_Num : Inport
  Choosing real control variables : MATLAB Function  TreatAsAtomicUnit=on
  Decenteralized Cooperaive Controller #4 : Subsystem
  Module to compute Consensus Error #4 : MATLAB Function  TreatAsAtomicUnit=on
  Mux : Mux  Inputs=2
  Variable change : MATLAB Function  TreatAsAtomicUnit=on
  u4 : Outport
  tag scope: E4_Cont=global, X4_Cont=global
  wires:
  Agent_Num/1 -> Module to compute Consensus Error #4/6(Agent_Num), Decenteralized Cooperaive Controller #4/1(Agent #)
  Decenteralized Cooperaive Controller #4/1(U4) -> Variable change/1(U), Choosing real control variables/1(U)
  [P_rel0_4] -> Module to compute Consensus Error #4/2(P_rel0)
  Module to compute Consensus Error #4/1(Ep) -> [E4_Cont]
  [P_rel_4] -> Module to compute Consensus Error #4/1(P_rel_all)
  Choosing real control variables/1(u) -> u4/1
  Variable change/1(X_mod) -> [X4_Cont]
  Mux/1 -> Variable change/2(X)
  [P4_hat] -> Mux/1
  [V4] -> Mux/2
  [V4] -> Module to compute Consensus Error #4/3(V_loc)
  [V0] -> Module to compute Consensus Error #4/4(V0)
  [V_all] -> Module to compute Consensus Error #4/5(V_all)

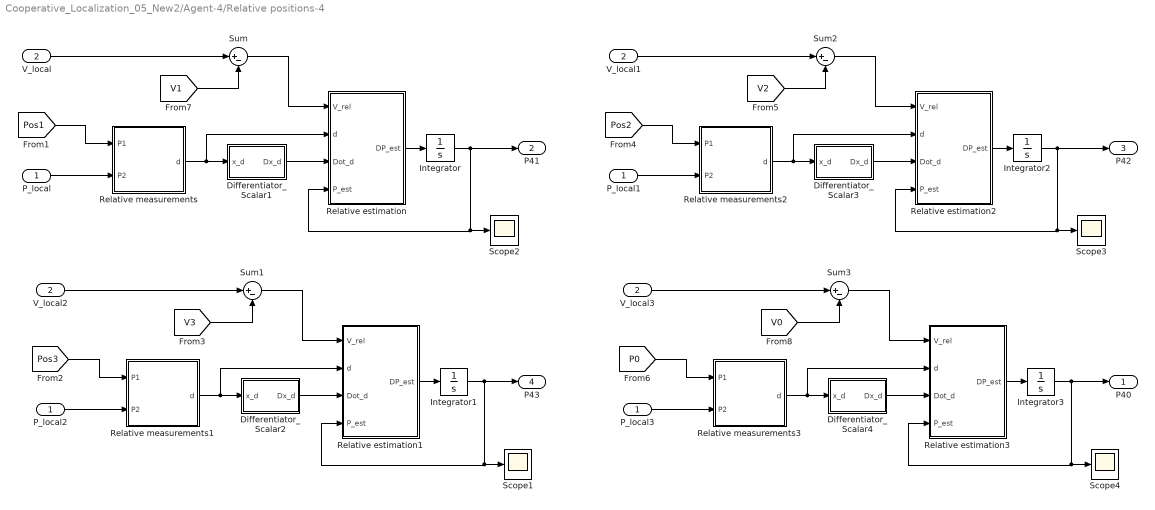
== system Cooperative_Localization_05_New2/Agent-4/Relative positions-4 ==
  P_local : Inport
  V_local : Inport  Port=2
  Differentiator_Scalar1 : Subsystem
  Differentiator_Scalar2 : Subsystem
  Differentiator_Scalar3 : Subsystem
  Differentiator_Scalar4 : Subsystem
  Integrator{,1..3} (4 alike) : Integrator  InitialCondition=zeros(2,1)
  P_local1 : InportShadow
  P_local2 : InportShadow
  P_local3 : InportShadow
  Relative estimation : MATLAB Function  TreatAsAtomicUnit=on
  Relative estimation1 : MATLAB Function  TreatAsAtomicUnit=on
  Relative estimation2 : MATLAB Function  TreatAsAtomicUnit=on
  Relative estimation3 : MATLAB Function  TreatAsAtomicUnit=on
  Relative measurements : MATLAB Function  TreatAsAtomicUnit=on
  Relative measurements1 : MATLAB Function  TreatAsAtomicUnit=on
  Relative measurements2 : MATLAB Function  TreatAsAtomicUnit=on
  Relative measurements3 : MATLAB Function  TreatAsAtomicUnit=on
  Scope{1..4} (4 alike) : Scope
  Sum{,1..3} (4 alike) : Sum  Inputs=|+-
  V_local1 : InportShadow  Port=2
  V_local2 : InportShadow  Port=2
  V_local3 : InportShadow  Port=2
  P40 : Outport
  P41 : Outport  Port=2
  P42 : Outport  Port=3
  P43 : Outport  Port=4
  wires:
  [P0] -> Relative measurements3/1(P1)
  [V0] -> Sum3/2
  Sum3/1 -> Relative estimation3/1(V_rel)
  V_local3/1 -> Sum3/1
  P_local3/1 -> Relative measurements3/2(P2)
  Integrator3/1 -> Relative estimation3/4(P_est), Scope4/1, P40/1
  Relative estimation3/1(DP_est) -> Integrator3/1
  Differentiator_Scalar4/1(Dx_d) -> Relative estimation3/3(Dot_d)
  Relative measurements3/1(d) -> Relative estimation3/2(d), Differentiator_Scalar4/1(x_d)
  [Pos2] -> Relative measurements2/1(P1)
  [V2] -> Sum2/2
  Sum2/1 -> Relative estimation2/1(V_rel)
  V_local1/1 -> Sum2/1
  P_local1/1 -> Relative measurements2/2(P2)
  Integrator2/1 -> Relative estimation2/4(P_est), Scope3/1, P42/1
  Relative estimation2/1(DP_est) -> Integrator2/1
  Differentiator_Scalar3/1(Dx_d) -> Relative estimation2/3(Dot_d)
  Relative measurements2/1(d) -> Relative estimation2/2(d), Differentiator_Scalar3/1(x_d)
  [Pos3] -> Relative measurements1/1(P1)
  [V3] -> Sum1/2
  Sum1/1 -> Relative estimation1/1(V_rel)
  V_local2/1 -> Sum1/1
  P_local2/1 -> Relative measurements1/2(P2)
  Integrator1/1 -> Relative estimation1/4(P_est), Scope1/1, P43/1
  Relative estimation1/1(DP_est) -> Integrator1/1
  Differentiator_Scalar2/1(Dx_d) -> Relative estimation1/3(Dot_d)
  Relative measurements1/1(d) -> Relative estimation1/2(d), Differentiator_Scalar2/1(x_d)
  [Pos1] -> Relative measurements/1(P1)
  [V1] -> Sum/2
  Sum/1 -> Relative estimation/1(V_rel)
  V_local/1 -> Sum/1
  P_local/1 -> Relative measurements/2(P2)
  Integrator/1 -> Relative estimation/4(P_est), Scope2/1, P41/1
  Relative estimation/1(DP_est) -> Integrator/1
  Differentiator_Scalar1/1(Dx_d) -> Relative estimation/3(Dot_d)
  Relative measurements/1(d) -> Relative estimation/2(d), Differentiator_Scalar1/1(x_d)

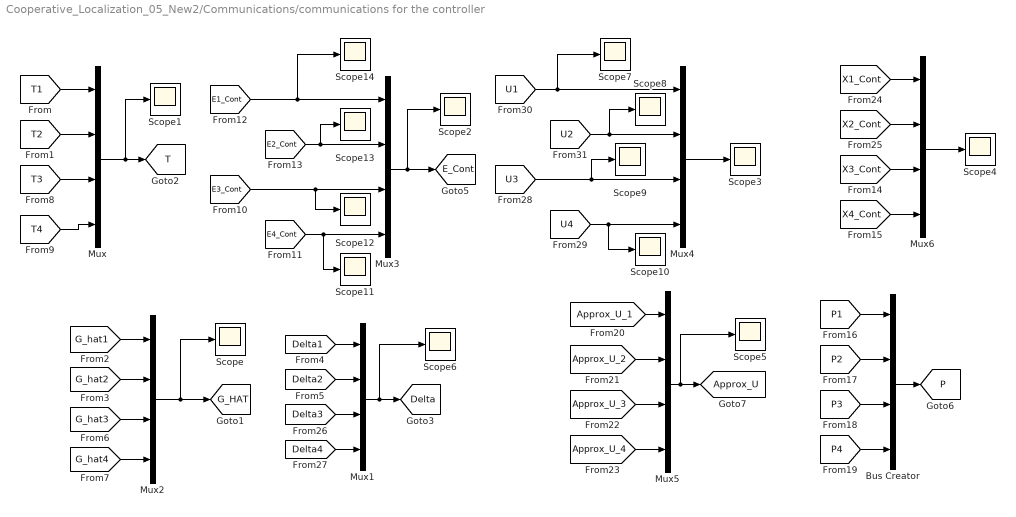
== system Cooperative_Localization_05_New2/Communications/communications for the controller ==
  Bus Creator : BusCreator  Inputs=4  OutDataTypeStr=Bus: P_bus
  Mux{,1..6} (7 alike) : Mux
  Scope{,1..14} (15 alike) : Scope
  tag scope: Approx_U=global, Delta=global, E_Cont=global, G_HAT=global, P=global, T=global
  wires:
  [T2] -> Mux/2
  [Delta1] -> Mux1/1
  [Delta2] -> Mux1/2
  Mux1/1 -> Scope6/1, [Delta]
  [T1] -> Mux/1
  [G_hat2] -> Mux2/2
  Mux2/1 -> Scope/1, [G_HAT]
  [G_hat1] -> Mux2/1
  Mux/1 -> Scope1/1, [T]
  [E2_Cont] -> Scope13/1, Mux3/2
  [E1_Cont] -> Scope14/1, Mux3/1
  Mux3/1 -> Scope2/1, [E_Cont]
  [P2] -> Bus Creator/2
  [P1] -> Bus Creator/1
  Bus Creator/1 -> [P]
  [Approx_U_2] -> Mux5/2
  [Approx_U_1] -> Mux5/1
  Mux5/1 -> [Approx_U], Scope5/1
  [G_hat3] -> Mux2/3
  [G_hat4] -> Mux2/4
  [T4] -> Mux/4
  [T3] -> Mux/3
  [E3_Cont] -> Scope12/1, Mux3/3
  [E4_Cont] -> Scope11/1, Mux3/4
  [P3] -> Bus Creator/3
  [P4] -> Bus Creator/4
  [Approx_U_3] -> Mux5/3
  [Approx_U_4] -> Mux5/4
  [Delta3] -> Mux1/3
  [Delta4] -> Mux1/4
  [U2] -> Scope8/1, Mux4/2
  [U1] -> Scope7/1, Mux4/1
  Mux4/1 -> Scope3/1
  [U3] -> Scope9/1, Mux4/3
  [U4] -> Scope10/1, Mux4/4
  [X2_Cont] -> Mux6/2
  [X1_Cont] -> Mux6/1
  Mux6/1 -> Scope4/1
  [X3_Cont] -> Mux6/3
  [X4_Cont] -> Mux6/4

== system Cooperative_Localization_05_New2/Leader/Agent-0 ==
  Control signal : Inport
  Clock : Clock
  Demux : Demux
  Demux1 : Demux  Outputs=2
  Integrator : Integrator  InitialCondition=[0;0;0;0]
  MATLAB Function : MATLAB Function  TreatAsAtomicUnit=on
  Memory1 : Memory  X0=zeros(2,1)
  Memory4 : Memory  X0=zeros(2,1)
  Mux : Mux  Inputs=2
  Mux1 : Mux  Inputs=2
  X0 : Outport
  P0 : Outport  Port=2
  V0 : Outport  Port=3
  wires:
  Control signal/1 -> Demux1/1
  Mux1/1 -> Memory1/1
  Mux/1 -> Memory4/1
  Memory4/1 -> P0/1
  Memory1/1 -> V0/1
  MATLAB Function/1(out) -> Integrator/1
  Integrator/1 -> Demux/1, X0/1
  Demux1/1 -> MATLAB Function/5(Ax)
  Demux1/2 -> MATLAB Function/6(Ay)
  Demux/3 -> Mux1/1, MATLAB Function/3(Vx)
  Demux/4 -> Mux1/2, MATLAB Function/4(Vy)
  Demux/1 -> Mux/1, MATLAB Function/1(Px)
  Demux/2 -> Mux/2, MATLAB Function/2(Py)
  Clock/1 -> MATLAB Function/7(t)

== system Cooperative_Localization_05_New2/Leader/Ali ==
  x : Inport
  xd : Inport  Port=2
  CARE : MATLAB Function  TreatAsAtomicUnit=on
  Differentiator : Subsystem
  Integrator : Integrator  InitialCondition=zeros(n_cont)
  Integrator1 : Integrator  InitialCondition=eye(n_cont)
  Integrator2 : Integrator  InitialCondition=zeros(n_cont,1)
  Integrator3 : Integrator  InitialCondition=zeros(n_cont,1)
  Memory : Memory  X0=zeros(m_cont,1)
  Scope{1..11} (11 alike) : Scope
  Sum : Sum  Inputs=|++
  g-Estimator : MATLAB Function  TreatAsAtomicUnit=on
  g-Estimator1 : MATLAB Function  TreatAsAtomicUnit=on
  main : MATLAB Function  TreatAsAtomicUnit=on
  variable change : MATLAB Function  TreatAsAtomicUnit=on
  u : Outport
  wires:
  xd/1 -> variable change/2(Xd)
  x/1 -> variable change/1(X)
  Integrator/1 -> Scope4/1, main/5(a_hat), CARE/2(a_hat), g-Estimator1/4(a_hat)
  Integrator1/1 -> main/4(P), g-Estimator/3(P), CARE/1(P), g-Estimator1/3(P), Scope5/1
  Sum/1 -> g-Estimator1/1(sigma), g-Estimator/1(sigma), Scope10/1, main/1(sigma)
  Differentiator/1(Dx_d) -> Scope8/1, main/3(Dy_d)
  g-Estimator1/1(Da_hat) -> Integrator/1
  variable change/1(x_mod) -> g-Estimator1/2(x), main/7(x), Scope11/1
  Integrator2/1 -> Scope2/1, main/6(g_hat), g-Estimator/2(g_hat)
  g-Estimator/1(Dg_hat) -> Integrator2/1, Scope3/1
  Integrator3/1 -> Sum/1, Scope6/1, main/2(zeta)
  Memory/1 -> Scope1/1, variable change/3(u)
  main/1(u) -> Memory/1, u/1
  CARE/1(DP) -> Integrator1/1
  variable change/2(xd_mod) -> Differentiator/1(x_d), Scope9/1
  variable change/3(e_mod) -> Integrator3/1, Scope7/1, Sum/2

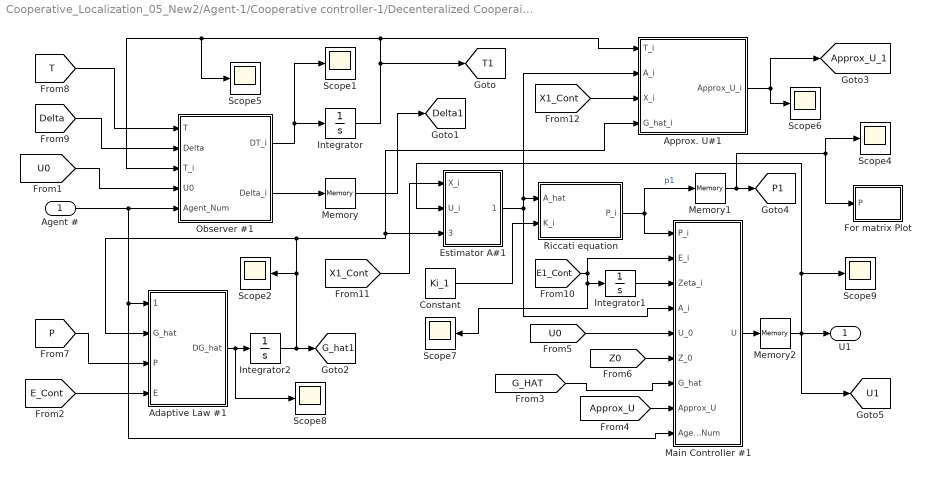
== system Cooperative_Localization_05_New2/Agent-1/Cooperative controller-1/Decenteralized Cooperaive Controller #1 ==
  Agent # : Inport
  Adaptive Law #1 : MATLAB Function  TreatAsAtomicUnit=on
  Approx. U#1 : MATLAB Function  TreatAsAtomicUnit=on
  Constant : Constant  Value=Ki_1
  Estimator A#1 : Subsystem
  For matrix Plot : Subsystem
  Integrator : Integrator  InitialCondition=zeros(n_cont,1)
  Integrator1 : Integrator  InitialCondition=zeros(n_cont,1)
  Integrator2 : Integrator  InitialCondition=zeros(t_cont,1)
  Main Controller #1 : MATLAB Function  TreatAsAtomicUnit=on
  Memory : Memory  X0=zeros(n_cont,1)
  Memory1 : Memory  X0=eye(n_cont)
  Memory2 : Memory  X0=zeros(m_cont,1)
  Observer #1 : MATLAB Function  TreatAsAtomicUnit=on
  Riccati equation : MATLAB Function  TreatAsAtomicUnit=on
  Scope{1..2,4..9} (8 alike) : Scope
  U1 : Outport
  tag scope: Approx_U_1=global, Delta1=global, G_hat1=global, P1=global, T1=global, U1=global
  wires:
  Memory/1 -> [Delta1]
  Agent #/1 -> Main Controller #1/9(Agent_Num), Adaptive Law #1/1(Agent_Num), Observer #1/5(Agent_Num)
  Observer #1/1(DT_i) -> Scope1/1, Integrator/1
  Observer #1/2(Delta_i) -> Memory/1
  [U0] -> Observer #1/4(U0)
  Adaptive Law #1/1(DG_hat) -> Scope8/1, Integrator2/1
  Integrator2/1 -> [G_hat1], Estimator A#1/3(G_hat_i), Approx. U#1/4(G_hat_i), Adaptive Law #1/2(G_hat), Scope2/1
  Integrator/1 -> Approx. U#1/1(T_i), Scope5/1, Observer #1/3(T_i), [T1]
  [Approx_U] -> Main Controller #1/8(Approx_U)
  [G_HAT] -> Main Controller #1/7(G_hat)
  [U0] -> Main Controller #1/5(U_0)
  [Z0] -> Main Controller #1/6(Z_0)
  Estimator A#1/1(A_hat_i) -> Main Controller #1/4(A_i), Riccati equation/1(A_hat), Approx. U#1/2(A_i)
  Riccati equation/1(P_i) -> Main Controller #1/1(P_i), Memory1/1  "p1"
  Main Controller #1/1(U) -> Memory2/1
  [P] -> Adaptive Law #1/3(P)
  [E_Cont] -> Adaptive Law #1/4(E)
  [T] -> Observer #1/1(T)
  [Delta] -> Observer #1/2(Delta)
  [E1_Cont] -> Main Controller #1/2(E_i), Integrator1/1, Scope7/1
  Integrator1/1 -> Main Controller #1/3(Zeta_i)
  [X1_Cont] -> Estimator A#1/1(X_i)
  [X1_Cont] -> Approx. U#1/3(X_i)
  Constant/1 -> Riccati equation/2(K_i)
  Memory2/1 -> [U1], Scope9/1, Estimator A#1/2(U_i), U1/1
  Memory1/1 -> For matrix Plot/1(P), Scope4/1, [P1]
  Approx. U#1/1(Approx_U_i) -> Scope6/1, [Approx_U_1]

== system Cooperative_Localization_05_New2/Agent-1/Relative positions-1/Differentiator_Scalar1 ==
  x_d : Inport
  Integrator : Integrator
  Integrator1 : Integrator
  Memory : Memory
  Scope : Scope
  Scope1 : Scope
  Sliding differentiator : MATLAB Function  TreatAsAtomicUnit=on
  Sliding differentiator1 : MATLAB Function  TreatAsAtomicUnit=on
  Sum : Sum  Inputs=|-+
  Dx_d : Outport
  wires:
  Sliding differentiator/1(u) -> Memory/1, Integrator1/1, Scope/1
  Integrator1/1 -> Sum/2
  Sum/1 -> Sliding differentiator1/1(e_inp), Sliding differentiator/2(e_inp), Scope1/1
  x_d/1 -> Sum/1
  Integrator/1 -> Sliding differentiator/1(u1)
  Sliding differentiator1/1(Du1) -> Integrator/1
  Memory/1 -> Dx_d/1

== system Cooperative_Localization_05_New2/Agent-1/Relative positions-1/Differentiator_Scalar2 ==
  x_d : Inport
  Integrator : Integrator
  Integrator1 : Integrator
  Memory : Memory
  Scope : Scope
  Scope1 : Scope
  Sliding differentiator : MATLAB Function  TreatAsAtomicUnit=on
  Sliding differentiator1 : MATLAB Function  TreatAsAtomicUnit=on
  Sum : Sum  Inputs=|-+
  Dx_d : Outport
  wires:
  Memory/1 -> Dx_d/1
  Sliding differentiator1/1(Du1) -> Integrator/1
  Integrator/1 -> Sliding differentiator/1(u1)
  x_d/1 -> Sum/1
  Sum/1 -> Scope1/1, Sliding differentiator/2(e_inp), Sliding differentiator1/1(e_inp)
  Integrator1/1 -> Sum/2
  Sliding differentiator/1(u) -> Scope/1, Integrator1/1, Memory/1

== system Cooperative_Localization_05_New2/Agent-1/Relative positions-1/Differentiator_Scalar3 ==
  x_d : Inport
  Integrator : Integrator
  Integrator1 : Integrator
  Memory : Memory
  Scope : Scope
  Scope1 : Scope
  Sliding differentiator : MATLAB Function  TreatAsAtomicUnit=on
  Sliding differentiator1 : MATLAB Function  TreatAsAtomicUnit=on
  Sum : Sum  Inputs=|-+
  Dx_d : Outport
  wires:
  Sliding differentiator/1(u) -> Memory/1, Integrator1/1, Scope/1
  Integrator1/1 -> Sum/2
  Sum/1 -> Sliding differentiator1/1(e_inp), Sliding differentiator/2(e_inp), Scope1/1
  x_d/1 -> Sum/1
  Integrator/1 -> Sliding differentiator/1(u1)
  Sliding differentiator1/1(Du1) -> Integrator/1
  Memory/1 -> Dx_d/1

== system Cooperative_Localization_05_New2/Agent-1/Relative positions-1/Differentiator_Scalar4 ==
  x_d : Inport
  Integrator : Integrator
  Integrator1 : Integrator
  Memory : Memory
  Scope : Scope
  Scope1 : Scope
  Sliding differentiator : MATLAB Function  TreatAsAtomicUnit=on
  Sliding differentiator1 : MATLAB Function  TreatAsAtomicUnit=on
  Sum : Sum  Inputs=|-+
  Dx_d : Outport
  wires:
  Sliding differentiator/1(u) -> Memory/1, Integrator1/1, Scope/1
  Integrator1/1 -> Sum/2
  Sum/1 -> Sliding differentiator1/1(e_inp), Sliding differentiator/2(e_inp), Scope1/1
  x_d/1 -> Sum/1
  Integrator/1 -> Sliding differentiator/1(u1)
  Sliding differentiator1/1(Du1) -> Integrator/1
  Memory/1 -> Dx_d/1

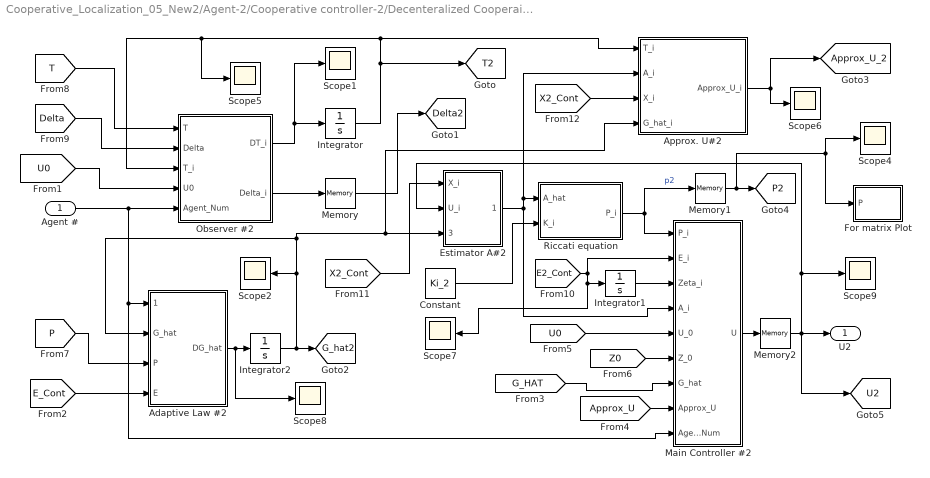
== system Cooperative_Localization_05_New2/Agent-2/Cooperative controller-2/Decenteralized Cooperaive Controller #2 ==
  Agent # : Inport
  Adaptive Law #2 : MATLAB Function  TreatAsAtomicUnit=on
  Approx. U#2 : MATLAB Function  TreatAsAtomicUnit=on
  Constant : Constant  Value=Ki_2
  Estimator A#2 : Subsystem
  For matrix Plot : Subsystem
  Integrator : Integrator  InitialCondition=zeros(n_cont,1)
  Integrator1 : Integrator  InitialCondition=zeros(n_cont,1)
  Integrator2 : Integrator  InitialCondition=zeros(t_cont,1)
  Main Controller #2 : MATLAB Function  TreatAsAtomicUnit=on
  Memory : Memory  X0=zeros(n_cont,1)
  Memory1 : Memory  X0=eye(n_cont)
  Memory2 : Memory  X0=zeros(m_cont,1)
  Observer #2 : MATLAB Function  TreatAsAtomicUnit=on
  Riccati equation : MATLAB Function  TreatAsAtomicUnit=on
  Scope{1..2,4..9} (8 alike) : Scope
  U2 : Outport
  tag scope: Approx_U_2=global, Delta2=global, G_hat2=global, P2=global, T2=global, U2=global
  wires:
  Memory/1 -> [Delta2]
  Agent #/1 -> Main Controller #2/9(Agent_Num), Adaptive Law #2/1(Agent_Num), Observer #2/5(Agent_Num)
  Observer #2/1(DT_i) -> Scope1/1, Integrator/1
  Observer #2/2(Delta_i) -> Memory/1
  [U0] -> Observer #2/4(U0)
  Adaptive Law #2/1(DG_hat) -> Scope8/1, Integrator2/1
  Integrator2/1 -> [G_hat2], Estimator A#2/3(G_hat_i), Approx. U#2/4(G_hat_i), Adaptive Law #2/2(G_hat), Scope2/1
  Integrator/1 -> Approx. U#2/1(T_i), Scope5/1, Observer #2/3(T_i), [T2]
  [Approx_U] -> Main Controller #2/8(Approx_U)
  [G_HAT] -> Main Controller #2/7(G_hat)
  [U0] -> Main Controller #2/5(U_0)
  [Z0] -> Main Controller #2/6(Z_0)
  Estimator A#2/1(A_hat_i) -> Main Controller #2/4(A_i), Riccati equation/1(A_hat), Approx. U#2/2(A_i)
  Riccati equation/1(P_i) -> Main Controller #2/1(P_i), Memory1/1  "p2"
  Main Controller #2/1(U) -> Memory2/1
  [P] -> Adaptive Law #2/3(P)
  [E_Cont] -> Adaptive Law #2/4(E)
  [T] -> Observer #2/1(T)
  [Delta] -> Observer #2/2(Delta)
  [E2_Cont] -> Main Controller #2/2(E_i), Integrator1/1, Scope7/1
  Integrator1/1 -> Main Controller #2/3(Zeta_i)
  [X2_Cont] -> Estimator A#2/1(X_i)
  [X2_Cont] -> Approx. U#2/3(X_i)
  Constant/1 -> Riccati equation/2(K_i)
  Memory2/1 -> [U2], Scope9/1, Estimator A#2/2(U_i), U2/1
  Memory1/1 -> For matrix Plot/1(P), Scope4/1, [P2]
  Approx. U#2/1(Approx_U_i) -> Scope6/1, [Approx_U_2]

== system Cooperative_Localization_05_New2/Agent-2/Relative positions-2/Differentiator_Scalar1 ==
  x_d : Inport
  Integrator : Integrator
  Integrator1 : Integrator
  Memory : Memory
  Scope : Scope
  Scope1 : Scope
  Sliding differentiator : MATLAB Function  TreatAsAtomicUnit=on
  Sliding differentiator1 : MATLAB Function  TreatAsAtomicUnit=on
  Sum : Sum  Inputs=|-+
  Dx_d : Outport
  wires:
  Memory/1 -> Dx_d/1
  Sliding differentiator1/1(Du1) -> Integrator/1
  Integrator/1 -> Sliding differentiator/1(u1)
  x_d/1 -> Sum/1
  Sum/1 -> Scope1/1, Sliding differentiator/2(e_inp), Sliding differentiator1/1(e_inp)
  Integrator1/1 -> Sum/2
  Sliding differentiator/1(u) -> Scope/1, Integrator1/1, Memory/1

== system Cooperative_Localization_05_New2/Agent-2/Relative positions-2/Differentiator_Scalar2 ==
  x_d : Inport
  Integrator : Integrator
  Integrator1 : Integrator
  Memory : Memory
  Scope : Scope
  Scope1 : Scope
  Sliding differentiator : MATLAB Function  TreatAsAtomicUnit=on
  Sliding differentiator1 : MATLAB Function  TreatAsAtomicUnit=on
  Sum : Sum  Inputs=|-+
  Dx_d : Outport
  wires:
  Sliding differentiator/1(u) -> Memory/1, Integrator1/1, Scope/1
  Integrator1/1 -> Sum/2
  Sum/1 -> Sliding differentiator1/1(e_inp), Sliding differentiator/2(e_inp), Scope1/1
  x_d/1 -> Sum/1
  Integrator/1 -> Sliding differentiator/1(u1)
  Sliding differentiator1/1(Du1) -> Integrator/1
  Memory/1 -> Dx_d/1

== system Cooperative_Localization_05_New2/Agent-2/Relative positions-2/Differentiator_Scalar3 ==
  x_d : Inport
  Integrator : Integrator
  Integrator1 : Integrator
  Memory : Memory
  Scope : Scope
  Scope1 : Scope
  Sliding differentiator : MATLAB Function  TreatAsAtomicUnit=on
  Sliding differentiator1 : MATLAB Function  TreatAsAtomicUnit=on
  Sum : Sum  Inputs=|-+
  Dx_d : Outport
  wires:
  Memory/1 -> Dx_d/1
  Sliding differentiator1/1(Du1) -> Integrator/1
  Integrator/1 -> Sliding differentiator/1(u1)
  x_d/1 -> Sum/1
  Sum/1 -> Scope1/1, Sliding differentiator/2(e_inp), Sliding differentiator1/1(e_inp)
  Integrator1/1 -> Sum/2
  Sliding differentiator/1(u) -> Scope/1, Integrator1/1, Memory/1

== system Cooperative_Localization_05_New2/Agent-2/Relative positions-2/Differentiator_Scalar4 ==
  x_d : Inport
  Integrator : Integrator
  Integrator1 : Integrator
  Memory : Memory
  Scope : Scope
  Scope1 : Scope
  Sliding differentiator : MATLAB Function  TreatAsAtomicUnit=on
  Sliding differentiator1 : MATLAB Function  TreatAsAtomicUnit=on
  Sum : Sum  Inputs=|-+
  Dx_d : Outport
  wires:
  Memory/1 -> Dx_d/1
  Sliding differentiator1/1(Du1) -> Integrator/1
  Integrator/1 -> Sliding differentiator/1(u1)
  x_d/1 -> Sum/1
  Sum/1 -> Scope1/1, Sliding differentiator/2(e_inp), Sliding differentiator1/1(e_inp)
  Integrator1/1 -> Sum/2
  Sliding differentiator/1(u) -> Scope/1, Integrator1/1, Memory/1

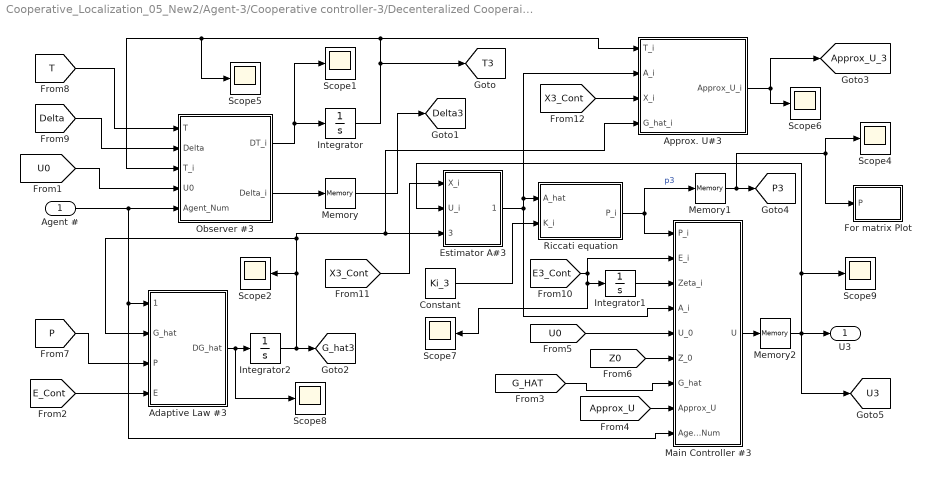
== system Cooperative_Localization_05_New2/Agent-3/Cooperative controller-3/Decenteralized Cooperaive Controller #3 ==
  Agent # : Inport
  Adaptive Law #3 : MATLAB Function  TreatAsAtomicUnit=on
  Approx. U#3 : MATLAB Function  TreatAsAtomicUnit=on
  Constant : Constant  Value=Ki_3
  Estimator A#3 : Subsystem
  For matrix Plot : Subsystem
  Integrator : Integrator  InitialCondition=zeros(n_cont,1)
  Integrator1 : Integrator  InitialCondition=zeros(n_cont,1)
  Integrator2 : Integrator  InitialCondition=zeros(t_cont,1)
  Main Controller #3 : MATLAB Function  TreatAsAtomicUnit=on
  Memory : Memory  X0=zeros(n_cont,1)
  Memory1 : Memory  X0=eye(n_cont)
  Memory2 : Memory  X0=zeros(m_cont,1)
  Observer #3 : MATLAB Function  TreatAsAtomicUnit=on
  Riccati equation : MATLAB Function  TreatAsAtomicUnit=on
  Scope{1..2,4..9} (8 alike) : Scope
  U3 : Outport
  tag scope: Approx_U_3=global, Delta3=global, G_hat3=global, P3=global, T3=global, U3=global
  wires:
  Memory/1 -> [Delta3]
  Agent #/1 -> Main Controller #3/9(Agent_Num), Adaptive Law #3/1(Agent_Num), Observer #3/5(Agent_Num)
  Observer #3/1(DT_i) -> Scope1/1, Integrator/1
  Observer #3/2(Delta_i) -> Memory/1
  [U0] -> Observer #3/4(U0)
  Adaptive Law #3/1(DG_hat) -> Scope8/1, Integrator2/1
  Integrator2/1 -> [G_hat3], Estimator A#3/3(G_hat_i), Approx. U#3/4(G_hat_i), Adaptive Law #3/2(G_hat), Scope2/1
  Integrator/1 -> Approx. U#3/1(T_i), Scope5/1, Observer #3/3(T_i), [T3]
  [Approx_U] -> Main Controller #3/8(Approx_U)
  [G_HAT] -> Main Controller #3/7(G_hat)
  [U0] -> Main Controller #3/5(U_0)
  [Z0] -> Main Controller #3/6(Z_0)
  Estimator A#3/1(A_hat_i) -> Main Controller #3/4(A_i), Riccati equation/1(A_hat), Approx. U#3/2(A_i)
  Riccati equation/1(P_i) -> Main Controller #3/1(P_i), Memory1/1  "p3"
  Main Controller #3/1(U) -> Memory2/1
  [P] -> Adaptive Law #3/3(P)
  [E_Cont] -> Adaptive Law #3/4(E)
  [T] -> Observer #3/1(T)
  [Delta] -> Observer #3/2(Delta)
  [E3_Cont] -> Main Controller #3/2(E_i), Integrator1/1, Scope7/1
  Integrator1/1 -> Main Controller #3/3(Zeta_i)
  [X3_Cont] -> Estimator A#3/1(X_i)
  [X3_Cont] -> Approx. U#3/3(X_i)
  Constant/1 -> Riccati equation/2(K_i)
  Memory2/1 -> [U3], Scope9/1, Estimator A#3/2(U_i), U3/1
  Memory1/1 -> For matrix Plot/1(P), Scope4/1, [P3]
  Approx. U#3/1(Approx_U_i) -> Scope6/1, [Approx_U_3]

== system Cooperative_Localization_05_New2/Agent-3/Relative positions-3/Differentiator_Scalar1 ==
  x_d : Inport
  Integrator : Integrator
  Integrator1 : Integrator
  Memory : Memory
  Scope : Scope
  Scope1 : Scope
  Sliding differentiator : MATLAB Function  TreatAsAtomicUnit=on
  Sliding differentiator1 : MATLAB Function  TreatAsAtomicUnit=on
  Sum : Sum  Inputs=|-+
  Dx_d : Outport
  wires:
  Sliding differentiator/1(u) -> Memory/1, Integrator1/1, Scope/1
  Integrator1/1 -> Sum/2
  Sum/1 -> Sliding differentiator1/1(e_inp), Sliding differentiator/2(e_inp), Scope1/1
  x_d/1 -> Sum/1
  Integrator/1 -> Sliding differentiator/1(u1)
  Sliding differentiator1/1(Du1) -> Integrator/1
  Memory/1 -> Dx_d/1

== system Cooperative_Localization_05_New2/Agent-3/Relative positions-3/Differentiator_Scalar2 ==
  x_d : Inport
  Integrator : Integrator
  Integrator1 : Integrator
  Memory : Memory
  Scope : Scope
  Scope1 : Scope
  Sliding differentiator : MATLAB Function  TreatAsAtomicUnit=on
  Sliding differentiator1 : MATLAB Function  TreatAsAtomicUnit=on
  Sum : Sum  Inputs=|-+
  Dx_d : Outport
  wires:
  Memory/1 -> Dx_d/1
  Sliding differentiator1/1(Du1) -> Integrator/1
  Integrator/1 -> Sliding differentiator/1(u1)
  x_d/1 -> Sum/1
  Sum/1 -> Scope1/1, Sliding differentiator/2(e_inp), Sliding differentiator1/1(e_inp)
  Integrator1/1 -> Sum/2
  Sliding differentiator/1(u) -> Scope/1, Integrator1/1, Memory/1

== system Cooperative_Localization_05_New2/Agent-3/Relative positions-3/Differentiator_Scalar3 ==
  x_d : Inport
  Integrator : Integrator
  Integrator1 : Integrator
  Memory : Memory
  Scope : Scope
  Scope1 : Scope
  Sliding differentiator : MATLAB Function  TreatAsAtomicUnit=on
  Sliding differentiator1 : MATLAB Function  TreatAsAtomicUnit=on
  Sum : Sum  Inputs=|-+
  Dx_d : Outport
  wires:
  Sliding differentiator/1(u) -> Memory/1, Integrator1/1, Scope/1
  Integrator1/1 -> Sum/2
  Sum/1 -> Sliding differentiator1/1(e_inp), Sliding differentiator/2(e_inp), Scope1/1
  x_d/1 -> Sum/1
  Integrator/1 -> Sliding differentiator/1(u1)
  Sliding differentiator1/1(Du1) -> Integrator/1
  Memory/1 -> Dx_d/1

== system Cooperative_Localization_05_New2/Agent-3/Relative positions-3/Differentiator_Scalar4 ==
  x_d : Inport
  Integrator : Integrator
  Integrator1 : Integrator
  Memory : Memory
  Scope : Scope
  Scope1 : Scope
  Sliding differentiator : MATLAB Function  TreatAsAtomicUnit=on
  Sliding differentiator1 : MATLAB Function  TreatAsAtomicUnit=on
  Sum : Sum  Inputs=|-+
  Dx_d : Outport
  wires:
  Sliding differentiator/1(u) -> Memory/1, Integrator1/1, Scope/1
  Integrator1/1 -> Sum/2
  Sum/1 -> Sliding differentiator1/1(e_inp), Sliding differentiator/2(e_inp), Scope1/1
  x_d/1 -> Sum/1
  Integrator/1 -> Sliding differentiator/1(u1)
  Sliding differentiator1/1(Du1) -> Integrator/1
  Memory/1 -> Dx_d/1
